simulink model "statechart2"  (R2016b)
settings: Solver=VariableStepAuto  StartTime=0.0  StopTime=10  MaxStep=0.05  RelTol=1e-3
libraries: dspindex x5
settings Model: Creator=larry  LastModifiedBy=larry

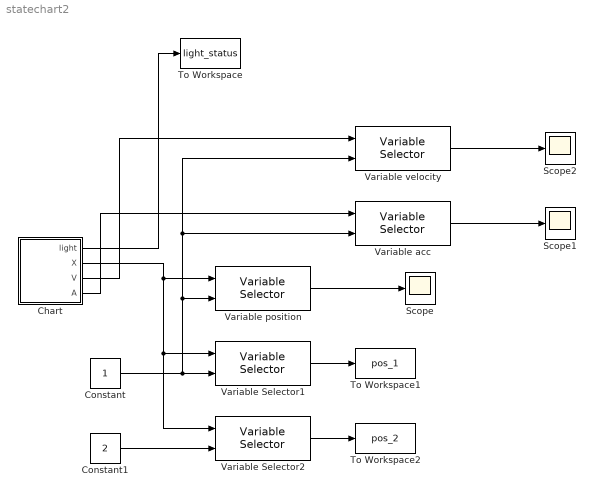
== system statechart2 ==
  Chart : Stateflow chart  TreatAsAtomicUnit=on
  Constant : Constant
  Constant1 : Constant  Value=2
  Scope : Scope
  Scope1 : Scope
  Scope2 : Scope
  To Workspace : ToWorkspace  VariableName=light_status  SampleTime=-1
  To Workspace1 : ToWorkspace  VariableName=pos_1  SampleTime=-1
  To Workspace2 : ToWorkspace  VariableName=pos_2  SampleTime=-1
  Variable Selector1 : dspindex/Variable Selector  NumInputs=1  rowsOrCols=Rows  IdxMode=Variable  Elements=[1 3]  ZerOneIdxMode=One-based  errmode=Clip Index  FillMode=on  FillValues=0
  Variable Selector2 : dspindex/Variable Selector  NumInputs=1  rowsOrCols=Rows  IdxMode=Variable  Elements=[1 3]  ZerOneIdxMode=One-based  errmode=Clip Index  FillMode=on  FillValues=0
  Variable acc : dspindex/Variable Selector  NumInputs=1  rowsOrCols=Columns  IdxMode=Variable  Elements=[1 3]  ZerOneIdxMode=One-based  errmode=Clip Index  FillMode=on  FillValues=0
  Variable position : dspindex/Variable Selector  NumInputs=1  rowsOrCols=Columns  IdxMode=Variable  Elements=[1 3]  ZerOneIdxMode=One-based  errmode=Clip Index  FillMode=on  FillValues=0
  Variable velocity : dspindex/Variable Selector  NumInputs=1  rowsOrCols=Columns  IdxMode=Variable  Elements=[1 3]  ZerOneIdxMode=One-based  errmode=Clip Index  FillMode=on  FillValues=0
  wires:
  Chart/1(light) -> To Workspace/1
  Chart/2(X) -> Variable Selector2/1, Variable Selector1/1, Variable position/1
  Constant/1 -> Variable Selector1/2, Variable acc/2, Variable velocity/2, Variable position/2
  Variable position/1 -> Scope/1
  Variable Selector1/1 -> To Workspace1/1
  Variable Selector2/1 -> To Workspace2/1
  Constant1/1 -> Variable Selector2/2
  Variable acc/1 -> Scope1/1
  Variable velocity/1 -> Scope2/1
  Chart/3(V) -> Variable velocity/1
  Chart/4(A) -> Variable acc/1

== stateflow chart statechart2/Chart ==
  state Light [parallel]
    settings: executionOrder=1
    state RED
      en:
      light = 1;
    state GREEN
      en:
      light = 0;
    (default) -> RED
    RED -> GREEN : after(2.5, sec)
    GREEN -> RED : after(2.5, sec)
  state Vehicle1 [parallel]
    settings: executionOrder=2
    state Straight
      state FreeDriving
        state AccFromStop
          en:
          A(this,:) = [A_MAX, 0];
          du:
          [X(this,:), V(this,:)] = accDrive(this, X, V, A);
        state Acc
          en:
          A(this,:) = [0.5*A_MAX, 0];
          du:
          [X(this,:), V(this,:)] = accDrive(this, X, V, A);
        state FixRate
          en:
          A(this,:) = [0, 0];
          V(this,:) = fixRate(this, V, V_MAX);
          du:
          X(this,:) = fixRateDrive(this, X, V);
        (default) -> (junction 71)
        (junction 71) -> AccFromStop [order 2]
        (junction 71) -> (junction 299) [order 1] : [~isStopped(this, V, D)]
        AccFromStop -> Acc : [reach(this, V, 3.0/5*V_MAX)]
        (junction 299) -> Acc [order 2]
        (junction 299) -> FixRate [order 1] : [reach(this, V, V_MAX)]
        Acc -> FixRate : [reach(this, V, V_MAX)]
      state Follow
        du:
        [X(this,:), V(this,:), A(this,:)] = ...
        followFrontCar(this, X, V, D, A_MAX);
      (default) -> FreeDriving
      FreeDriving -> Follow : [hasFrontCar(this, X, D)]
      Follow -> FreeDriving : [~hasFrontCar(this, X, D)]
    state SlowToStop
      state SlowDown
        en:
        A(this,:) = reqAcc(this, X, V, A_MAX, stopline);
        du:
        [X(this,:), V(this,:)] = accDrive(this, X, V, A);
      state Stopped
        en:
        A(this,:) = [0, 0];
        V(this,:) = [0, 0];
      (default) -> SlowDown
      SlowDown -> Stopped : [isStopped(this, V, D)]
    (default) -> Straight
    SlowToStop -> Straight : [lightGreen()]
    Straight -> SlowToStop : [stoppedByRed(this, X, V, D, A_MAX, stopline)]
  data: self function_input; Xi function_input; Vi function_input; amax function_input; a function_output; inter function_input; self function_input; Vi function_input; Di function_input; res function_output; self function_input; res function_output; Xi function_input; Di function_input; self function_input; Xi function_input; Vi function_input; x function_output; self function_input; res function_output; Xi function_input; Di function_input; inter function_input; self function_input; Vi function_input; s function_input; v function_output; self function_input; Xi function_input; Vi function_input; Ai function_input; x function_output; v function_output; self function_input; res function_output; Xi function_input; Vi function_input; Di function_input; amax function_input; inter function_input; this constant uint8 =1; V_MAX constant double size=1 =2.5; A_MAX constant double size=1 =3; self function_input; Xi function_input; Vi function_input; amax function_input; res function_output; inter function_input; self function_input; Vi function_input; vmax function_input; res function_output; self function_input; Xi function_input; Vi function_input; Di function_input; x function_output; v function_output; amax function_input; a function_output; res function_output; dt constant double size=1 =0.05; stopline constant double size=[1 2] =[-1 -0.5]; light output; WORLD_SIZE constant double size=1 =8; X output size=[2, 2] =[-5, -0.5; 3, -0.5]; D local size=[2, 2] =[1, 0; 1, 0]; SAFE_DIST constant double size=1 =1; V output size=[2, 2] =[0, 0; 0, 0]; A output size=[2, 2] =[0, 0; 0, 0]
  function a = reqAcc(self, Xi, Vi, amax, inter):
    | function a = reqAcc(self, Xi, Vi, amax, inter)
    | 
    | x = Xi(self, :);
    | v = Vi(self, :);
    | 
    | dx = inter - x;
    | % add safe distance
    | dist = norm(dx) - SAFE_DIST;
    | if dot(dx, v) < 0
    |     a = [0 0];
    | else
    |     vnorm = norm(v);
    |     reverse = v/vnorm*(-1);
    |     a = reverse*vnorm*vnorm/2/dist;
    |     anorm = norm(a);
    |     if(anorm >= amax)
    |         a = a/anorm*amax;
    |     end
    | end
  function res = isStopped(self, Vi, Di):
    | function res = isStopped(self, Vi, Di)
    | 
    | v = Vi(self,:);
    | d = Di(self,:);
    | res = false;
    | if(dot(v, d) <= 0)
    |     res = true;
    | end
    | if norm(v) <= 1e-3
    |     res = true;
    | end
  function res = hasFrontCar(self, Xi, Di):
    | function res = hasFrontCar(self, Xi, Di)
    | 
    | dX = zeros(size(Xi, 1));
    | x = Xi(self,:);
    | d = Di(self,:);
    | for k=1:length(dX)
    |     dX(k) = dot(Xi(k,:) - x, d);
    |     if dX(k) < 0
    |         dX(k) = dX(k) + WORLD_SIZE;
    |     end
    | end
    | 
    | dist = min(dX(dX > 0));
    | res = (dist < 2*SAFE_DIST);
    | 
    | % res = false;
  function x = fixRateDrive(self, Xi, Vi):
    | function x = fixRateDrive(self, Xi, Vi)
    |  
    | x = Xi(self, :);
    | v = Vi(self, :);
    | 
    | x = x + v * dt;
    | % a rounded world
    | if x(1) > WORLD_SIZE
    |     x(1) = -WORLD_SIZE;
    | elseif x(1) < -WORLD_SIZE
    |     x(1) = WORLD_SIZE;
    | end
  function res = closeToInter(self, Xi, Di, inter):
    | function res = closeToInter(self, Xi, Di, inter)
    | 
    | x = Xi(self, :);
    | d = Di(self, :);
    | 
    | inner = dot(inter - x, d);
    | if inner >= 0 && inner <= 2.5
    |     res = true;
    | else
    |     res = false;
    | end
  function v = fixRate(self, Vi, s):
    | function v = fixRate(self, Vi, s)
    |  
    | v = Vi(self, :);
    | if norm(v) < 1e-6
    |     v = [0 0];
    | else
    |     v = v/norm(v)*s;
    | end
  function [x, v] = accDrive(self, Xi, Vi, Ai):
    | function [x, v] = accDrive(self, Xi, Vi, Ai)
    | 
    | x = Xi(self, :);
    | v = Vi(self, :);
    | a = Ai(self, :);
    | 
    | x = x + v * dt + 0.5 * a * dt * dt;
    | v = v + a * dt;
    | 
    | if x(1) > WORLD_SIZE
    |     x(1) = -WORLD_SIZE;
    | elseif x(1) < -WORLD_SIZE
    |     x(1) = WORLD_SIZE;
    | end
  function res = stoppedByRed(self, Xi, Vi, Di, amax, inter):
    | function res = stoppedByRed(self, Xi, Vi, Di, amax, inter)
    | 
    | if closeToInter(self, Xi, Di, inter) && ...
    |         isStoppable(self, Xi, Vi, amax, inter) && ...
    |         in(Light.RED)
    |     res = true;
    | else
    |     res = false;
    | end
  function res = isStoppable(self, Xi, Vi, amax, inter):
    | function res = isStoppable(self, Xi, Vi, amax, inter)
    | 
    | x = Xi(self, :);
    | v = Vi(self, :);
    | dist = norm(inter - x);
    | 
    | vnorm = norm(v);
    | brake_dist = vnorm*vnorm/2.0/amax;
    | res = (brake_dist <= dist);
  function res = reach(self, Vi, vmax):
    | function res = reach(self, Vi, vmax)
    | 
    | res = false;
    | if norm(Vi(self, :)) >= vmax
    |     res = true;
    | end
  function [x, v, a] = followFrontCar(self, Xi, Vi, Di, amax):
    | function [x, v, a] = followFrontCar(self, Xi, Vi, Di, amax)
    | 
    | dX = zeros(size(Xi, 1));
    | x = Xi(self,:);
    | v = Vi(self,:);
    | d = Di(self,:);
    | a = [0, 0];
    | 
    | for k=1:length(dX)
    |     dX(k) = dot(Xi(k,:) - x, d);
    |     if dX(k) < 0
    |         dX(k) = dX(k) + WORLD_SIZE;
    |     end
    | end
    | 
    | dist = min(dX(dX > 0));
    | idx = find(dX == dist);
    | 
    | % there must be only one vehicle in front of target agent
    | assert(length(idx) == 1);
    | vo = Vi(idx(1), :);
    | 
    | if dist < 2*SAFE_DIST
    |     ar = (vo - v) / dt;
    |     arnorm = norm(ar);
    |     if arnorm > amax
    |         ar = ar/arnorm * amax;
    |         x = x + v * dt + 0.5 * ar * dt * dt;
    |         v = v + ar * dt;
    |     else
    |         x = x + (v + vo) * dt / 2;
    |         v = vo;
    |     end
    |     a = ar;
    | else
    |     x = x + v * dt;
    | end
  function res = lightGreen:
    | function res = lightGreen
    | 
    | if in(Light.GREEN)
    |     res = true;
    | else 
    |     res = false;
    | end
